simulink model "Lab2"  (R2018a)
settings: Solver=VariableStepAuto  StartTime=0.0  StopTime=2  RelTol=1e-3
libraries: simulink x5
settings Model: Creator=libingra  LastModifiedBy=libingra

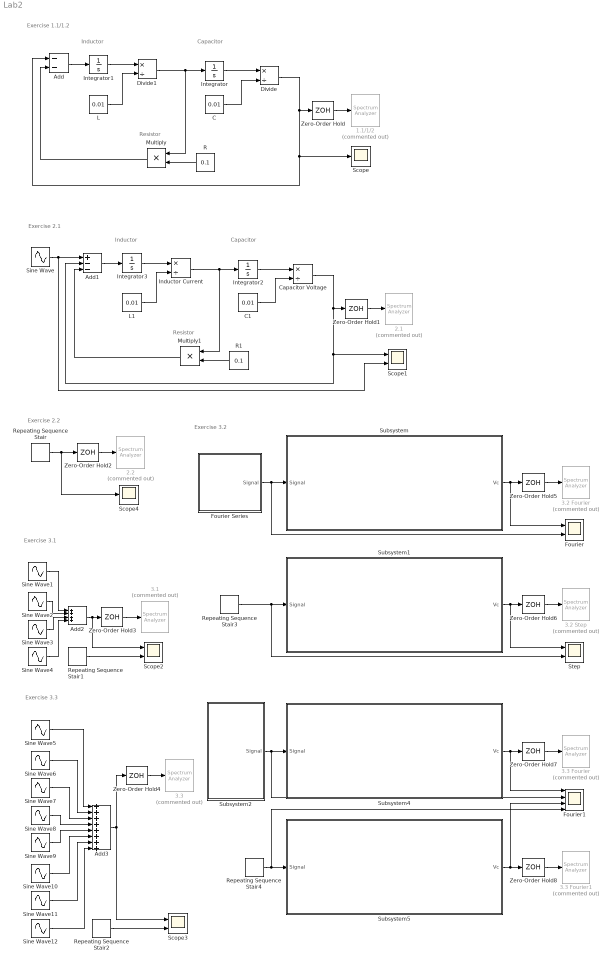
== system Lab2 ==
  note: Exercise 3.3
  note: Exercise 3.2
  note: Exercise 3.1
  note: Exercise 2.1
  note: Exercise 1.1/1.2
  note: Exercise 2.2
  note: Resistor
  note: Capacitor
  note: Inductor
  note: Inductor
  note: Capacitor
  note: Resistor
  1.1/1/2 : SpectrumAnalyzer  Commented=on
  2.1 : SpectrumAnalyzer  Commented=on
  2.2 : SpectrumAnalyzer  Commented=on
  3.1 : SpectrumAnalyzer  Commented=on
  3.2 Fourier : SpectrumAnalyzer  Commented=on
  3.2 Step : SpectrumAnalyzer  Commented=on
  3.3 : SpectrumAnalyzer  Commented=on
  3.3 Fourier : SpectrumAnalyzer  Commented=on
  3.3 Fourier1 : SpectrumAnalyzer  Commented=on
  Add : Sum  Inputs=--
  Add1 : Sum  Inputs=+--
  Add2 : Sum  Inputs=++++
  Add3 : Sum  Inputs=++++++++
  C : Constant  Value=0.01
  C1 : Constant  Value=0.01
  Capacitor Voltage : Product  Inputs=*/
  Divide : Product  Inputs=*/
  Divide1 : Product  Inputs=*/
  Fourier : Scope  NumInputPorts=2
  Fourier Series : Subsystem
  Fourier1 : Scope  NumInputPorts=4
  Inductor Current : Product  Inputs=*/
  Integrator : Integrator  InitialCondition=0.1
  Integrator1 : Integrator  InitialCondition=0.1
  Integrator2 : Integrator
  Integrator3 : Integrator
  L : Constant  Value=0.01
  L1 : Constant  Value=0.01
  Multiply : Product
  Multiply1 : Product
  R : Constant  Value=0.1
  R1 : Constant  Value=0.1
  Repeating Sequence Stair{,1..4} (5 alike) : simulink/Sources/Repeating Sequence Stair  OutValues=[1 -1].'  tsamp=1/64  OutMin=[]  OutMax=[]  OutDataTypeStr=double  OutputDataTypeScalingMode=double  OutDataType=fixdt(0,8)  ConRadixGroup=Best Precision: Vector-wise  OutScaling=2^-12
  Scope : Scope
  Scope1 : Scope  NumInputPorts=2
  Scope2 : Scope  NumInputPorts=2
  Scope3 : Scope  NumInputPorts=2
  Scope4 : Scope
  Sine Wave : Sin  Frequency=100*2  SampleTime=0
  Sine Wave1 : Sin  Amplitude=4/(1*pi)  Frequency=64*pi*1  SampleTime=0
  Sine Wave10 : Sin  Amplitude=4/(11*pi)  Frequency=64*pi*11  SampleTime=0
  Sine Wave11 : Sin  Amplitude=4/(13*pi)  Frequency=64*pi*13  SampleTime=0
  Sine Wave12 : Sin  Amplitude=4/(15*pi)  Frequency=64*pi*15  SampleTime=0
  Sine Wave2 : Sin  Amplitude=4/(3*pi)  Frequency=64*pi*3  SampleTime=0
  Sine Wave3 : Sin  Amplitude=4/(5*pi)  Frequency=64*pi*5  SampleTime=0
  Sine Wave4 : Sin  Amplitude=4/(7*pi)  Frequency=64*pi*7  SampleTime=0
  Sine Wave5 : Sin  Amplitude=4/(1*pi)  Frequency=64*pi*1  SampleTime=0
  Sine Wave6 : Sin  Amplitude=4/(3*pi)  Frequency=64*pi*3  SampleTime=0
  Sine Wave7 : Sin  Amplitude=4/(5*pi)  Frequency=64*pi*5  SampleTime=0
  Sine Wave8 : Sin  Amplitude=4/(7*pi)  Frequency=64*pi*7  SampleTime=0
  Sine Wave9 : Sin  Amplitude=4/(9*pi)  Frequency=64*pi*9  SampleTime=0
  Step : Scope  NumInputPorts=2
  Subsystem : Subsystem
  Subsystem1 : Subsystem
  Subsystem2 : Subsystem
  Subsystem4 : Subsystem
  Subsystem5 : Subsystem
  Zero-Order Hold{,1..8} (9 alike) : ZeroOrderHold  SampleTime=2^-10
  wires:
  L/1 -> Divide1/2
  Integrator1/1 -> Divide1/1
  Add/1 -> Integrator1/1
  Integrator/1 -> Divide/1
  C/1 -> Divide/2
  Divide1/1 -> Multiply/1, Integrator/1
  R/1 -> Multiply/2
  Multiply/1 -> Add/2
  Divide/1 -> Zero-Order Hold/1, Scope/1, Add/1
  Zero-Order Hold/1 -> 1.1/1/2/1
  Multiply1/1 -> Add1/3
  R1/1 -> Multiply1/2
  Inductor Current/1 -> Multiply1/1, Integrator2/1
  L1/1 -> Inductor Current/2
  Add1/1 -> Integrator3/1
  C1/1 -> Capacitor Voltage/2
  Integrator3/1 -> Inductor Current/1
  Integrator2/1 -> Capacitor Voltage/1
  Zero-Order Hold1/1 -> 2.1/1
  Capacitor Voltage/1 -> Zero-Order Hold1/1, Add1/2, Scope1/1
  Sine Wave/1 -> Scope1/2, Add1/1
  Zero-Order Hold2/1 -> 2.2/1
  Repeating Sequence Stair/1 -> Scope4/1, Zero-Order Hold2/1
  Sine Wave1/1 -> Add2/1
  Sine Wave2/1 -> Add2/2
  Sine Wave3/1 -> Add2/3
  Sine Wave4/1 -> Add2/4
  Add2/1 -> Scope2/1, Zero-Order Hold3/1
  Repeating Sequence Stair1/1 -> Scope2/2
  Zero-Order Hold3/1 -> 3.1/1
  Add3/1 -> Scope3/1, Zero-Order Hold4/1
  Repeating Sequence Stair2/1 -> Scope3/2
  Sine Wave8/1 -> Add3/4
  Zero-Order Hold4/1 -> 3.3/1
  Sine Wave7/1 -> Add3/3
  Sine Wave6/1 -> Add3/2
  Sine Wave5/1 -> Add3/1
  Sine Wave9/1 -> Add3/5
  Sine Wave10/1 -> Add3/6
  Sine Wave11/1 -> Add3/7
  Sine Wave12/1 -> Add3/8
  Fourier Series/1(Signal) -> Fourier/2, Subsystem/1(Signal)
  Zero-Order Hold5/1 -> 3.2 Fourier/1
  Subsystem/1(Vc) -> Zero-Order Hold5/1, Fourier/1
  Zero-Order Hold6/1 -> 3.2 Step/1
  Subsystem1/1(Vc) -> Zero-Order Hold6/1, Step/1
  Repeating Sequence Stair3/1 -> Step/2, Subsystem1/1(Signal)
  Zero-Order Hold7/1 -> 3.3 Fourier/1
  Subsystem4/1(Vc) -> Zero-Order Hold7/1, Fourier1/1
  Subsystem2/1(Signal) -> Subsystem4/1(Signal), Fourier1/2
  Zero-Order Hold8/1 -> 3.3 Fourier1/1
  Subsystem5/1(Vc) -> Zero-Order Hold8/1, Fourier1/3
  Repeating Sequence Stair4/1 -> Fourier1/4, Subsystem5/1(Signal)

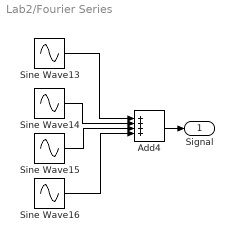
== system Lab2/Fourier Series ==
  Add4 : Sum  Inputs=++++
  Sine Wave13 : Sin  Amplitude=4/(1*pi)  Frequency=64*pi*1  SampleTime=0
  Sine Wave14 : Sin  Amplitude=4/(3*pi)  Frequency=64*pi*3  SampleTime=0
  Sine Wave15 : Sin  Amplitude=4/(5*pi)  Frequency=64*pi*5  SampleTime=0
  Sine Wave16 : Sin  Amplitude=4/(7*pi)  Frequency=64*pi*7  SampleTime=0
  Signal : Outport
  wires:
  Add4/1 -> Signal/1
  Sine Wave13/1 -> Add4/1
  Sine Wave14/1 -> Add4/2
  Sine Wave15/1 -> Add4/3
  Sine Wave16/1 -> Add4/4

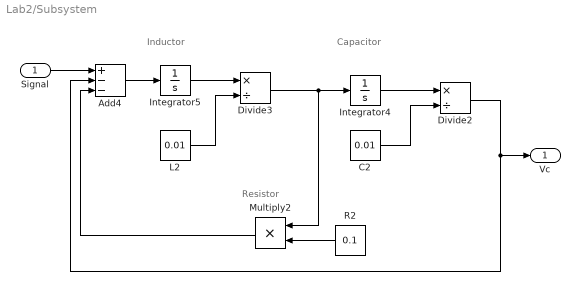
== system Lab2/Subsystem ==
  note: Inductor
  note: Resistor
  note: Capacitor
  Signal : Inport
  Add4 : Sum  Inputs=+--
  C2 : Constant  Value=0.01
  Divide2 : Product  Inputs=*/
  Divide3 : Product  Inputs=*/
  Integrator4 : Integrator  InitialCondition=0.1
  Integrator5 : Integrator  InitialCondition=0.1
  L2 : Constant  Value=0.01
  Multiply2 : Product
  R2 : Constant  Value=0.1
  Vc : Outport
  wires:
  Integrator5/1 -> Divide3/1
  Divide3/1 -> Multiply2/1, Integrator4/1
  R2/1 -> Multiply2/2
  L2/1 -> Divide3/2
  Signal/1 -> Add4/1
  Add4/1 -> Integrator5/1
  Integrator4/1 -> Divide2/1
  Divide2/1 -> Add4/2, Vc/1
  Multiply2/1 -> Add4/3
  C2/1 -> Divide2/2

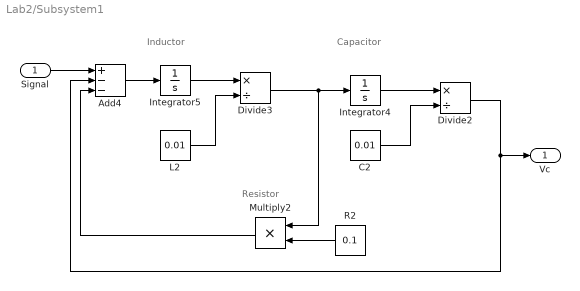
== system Lab2/Subsystem1 ==
  note: Inductor
  note: Resistor
  note: Capacitor
  Signal : Inport
  Add4 : Sum  Inputs=+--
  C2 : Constant  Value=0.01
  Divide2 : Product  Inputs=*/
  Divide3 : Product  Inputs=*/
  Integrator4 : Integrator  InitialCondition=0.1
  Integrator5 : Integrator  InitialCondition=0.1
  L2 : Constant  Value=0.01
  Multiply2 : Product
  R2 : Constant  Value=0.1
  Vc : Outport
  wires:
  Integrator5/1 -> Divide3/1
  Divide3/1 -> Multiply2/1, Integrator4/1
  R2/1 -> Multiply2/2
  L2/1 -> Divide3/2
  Signal/1 -> Add4/1
  Add4/1 -> Integrator5/1
  Integrator4/1 -> Divide2/1
  Divide2/1 -> Add4/2, Vc/1
  Multiply2/1 -> Add4/3
  C2/1 -> Divide2/2

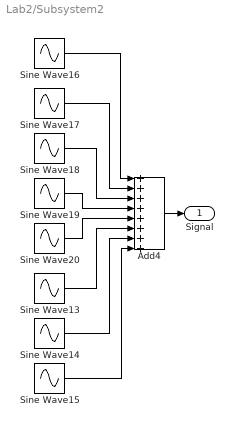
== system Lab2/Subsystem2 ==
  Add4 : Sum  Inputs=++++++++
  Sine Wave13 : Sin  Amplitude=4/(11*pi)  Frequency=64*pi*11  SampleTime=0
  Sine Wave14 : Sin  Amplitude=4/(13*pi)  Frequency=64*pi*13  SampleTime=0
  Sine Wave15 : Sin  Amplitude=4/(15*pi)  Frequency=64*pi*15  SampleTime=0
  Sine Wave16 : Sin  Amplitude=4/(1*pi)  Frequency=64*pi*1  SampleTime=0
  Sine Wave17 : Sin  Amplitude=4/(3*pi)  Frequency=64*pi*3  SampleTime=0
  Sine Wave18 : Sin  Amplitude=4/(5*pi)  Frequency=64*pi*5  SampleTime=0
  Sine Wave19 : Sin  Amplitude=4/(7*pi)  Frequency=64*pi*7  SampleTime=0
  Sine Wave20 : Sin  Amplitude=4/(9*pi)  Frequency=64*pi*9  SampleTime=0
  Signal : Outport
  wires:
  Sine Wave17/1 -> Add4/2
  Sine Wave13/1 -> Add4/6
  Sine Wave15/1 -> Add4/8
  Sine Wave14/1 -> Add4/7
  Sine Wave20/1 -> Add4/5
  Add4/1 -> Signal/1
  Sine Wave19/1 -> Add4/4
  Sine Wave18/1 -> Add4/3
  Sine Wave16/1 -> Add4/1

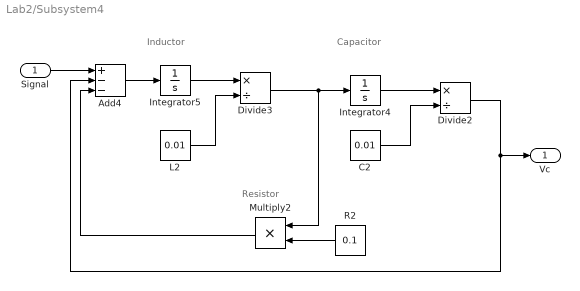
== system Lab2/Subsystem4 ==
  note: Inductor
  note: Resistor
  note: Capacitor
  Signal : Inport
  Add4 : Sum  Inputs=+--
  C2 : Constant  Value=0.01
  Divide2 : Product  Inputs=*/
  Divide3 : Product  Inputs=*/
  Integrator4 : Integrator  InitialCondition=0.1
  Integrator5 : Integrator  InitialCondition=0.1
  L2 : Constant  Value=0.01
  Multiply2 : Product
  R2 : Constant  Value=0.1
  Vc : Outport
  wires:
  Integrator5/1 -> Divide3/1
  Divide3/1 -> Multiply2/1, Integrator4/1
  R2/1 -> Multiply2/2
  L2/1 -> Divide3/2
  Signal/1 -> Add4/1
  Add4/1 -> Integrator5/1
  Integrator4/1 -> Divide2/1
  Divide2/1 -> Add4/2, Vc/1
  Multiply2/1 -> Add4/3
  C2/1 -> Divide2/2

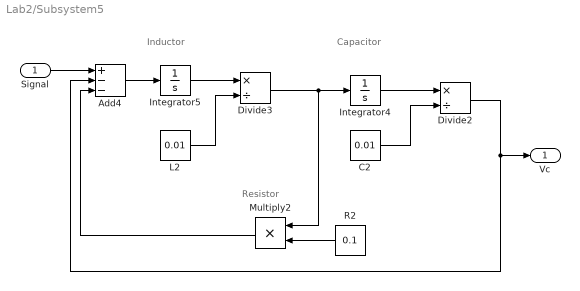
== system Lab2/Subsystem5 ==
  note: Inductor
  note: Resistor
  note: Capacitor
  Signal : Inport
  Add4 : Sum  Inputs=+--
  C2 : Constant  Value=0.01
  Divide2 : Product  Inputs=*/
  Divide3 : Product  Inputs=*/
  Integrator4 : Integrator  InitialCondition=0.1
  Integrator5 : Integrator  InitialCondition=0.1
  L2 : Constant  Value=0.01
  Multiply2 : Product
  R2 : Constant  Value=0.1
  Vc : Outport
  wires:
  Integrator5/1 -> Divide3/1
  Divide3/1 -> Multiply2/1, Integrator4/1
  R2/1 -> Multiply2/2
  L2/1 -> Divide3/2
  Signal/1 -> Add4/1
  Add4/1 -> Integrator5/1
  Integrator4/1 -> Divide2/1
  Divide2/1 -> Add4/2, Vc/1
  Multiply2/1 -> Add4/3
  C2/1 -> Divide2/2
